simulink model "Enable_Subsystem"  (R2024b)
settings: Solver=VariableStepAuto  StartTime=0.0  StopTime=10.0  RelTol=1e-3
settings Model: Creator=Ahmad  LastModifiedBy=Ahmad

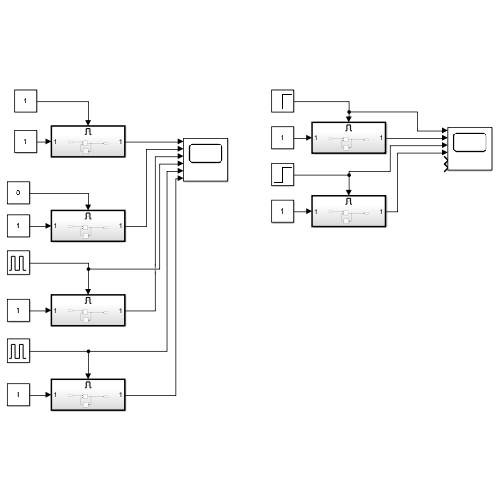
[thumbnail: Simulink's stored preview of the top-level diagram]
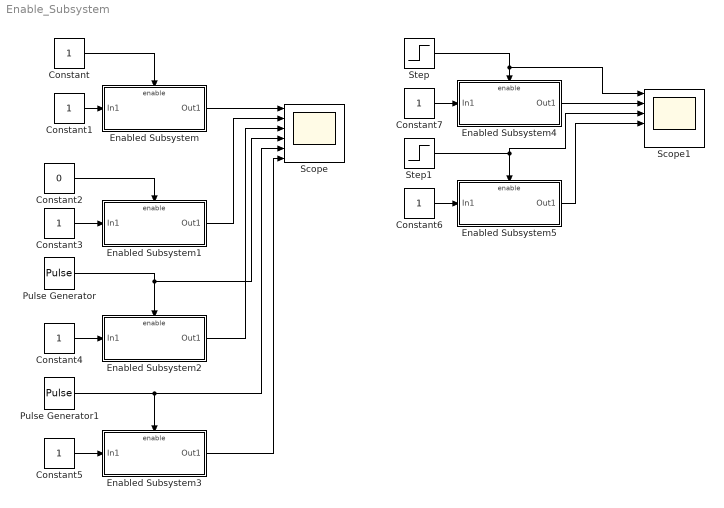
== system Enable_Subsystem ==
  Constant{,1,3..7} (7 alike) : Constant
  Constant2 : Constant  Value=0
  Enabled Subsystem : Subsystem  TreatAsAtomicUnit=on
  Enabled Subsystem1 : Subsystem  TreatAsAtomicUnit=on
  Enabled Subsystem2 : Subsystem  TreatAsAtomicUnit=on
  Enabled Subsystem3 : Subsystem  TreatAsAtomicUnit=on
  Enabled Subsystem4 : Subsystem  TreatAsAtomicUnit=on
  Enabled Subsystem5 : Subsystem  TreatAsAtomicUnit=on
  Pulse Generator : DiscretePulseGenerator  PulseType=Time based  Period=1  PulseWidth=50
  Pulse Generator1 : DiscretePulseGenerator  PulseType=Time based  Period=1  PulseWidth=50
  Scope : Scope  NumInputPorts=6
  Scope1 : Scope  NumInputPorts=6
  Step : Step  SampleTime=0
  Step1 : Step  Before=-2  After=0  SampleTime=0
  wires:
  Enabled Subsystem/1(Out1) -> Scope/1
  Constant/1 -> Enabled Subsystem/Enable
  Constant1/1 -> Enabled Subsystem/1(In1)
  Constant3/1 -> Enabled Subsystem1/1(In1)
  Constant2/1 -> Enabled Subsystem1/Enable
  Enabled Subsystem1/1(Out1) -> Scope/2
  Constant4/1 -> Enabled Subsystem2/1(In1)
  Pulse Generator/1 -> Enabled Subsystem2/Enable, Scope/4
  Enabled Subsystem2/1(Out1) -> Scope/3
  Pulse Generator1/1 -> Scope/5, Enabled Subsystem3/Enable
  Constant5/1 -> Enabled Subsystem3/1(In1)
  Enabled Subsystem3/1(Out1) -> Scope/6
  Constant7/1 -> Enabled Subsystem4/1(In1)
  Step/1 -> Scope1/1, Enabled Subsystem4/Enable
  Enabled Subsystem4/1(Out1) -> Scope1/2
  Constant6/1 -> Enabled Subsystem5/1(In1)
  Step1/1 -> Scope1/3, Enabled Subsystem5/Enable
  Enabled Subsystem5/1(Out1) -> Scope1/4

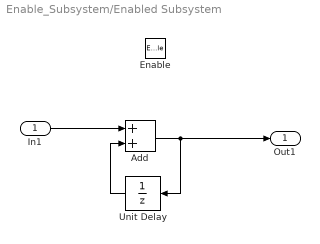
== system Enable_Subsystem/Enabled Subsystem ==
  In1 : Inport
  Enable : EnablePort
  Add : Sum
  Unit Delay : UnitDelay  SampleTime=-1  HasFrameUpgradeWarning=on
  Out1 : Outport
  wires:
  In1/1 -> Add/1
  Add/1 -> Unit Delay/1, Out1/1
  Unit Delay/1 -> Add/2

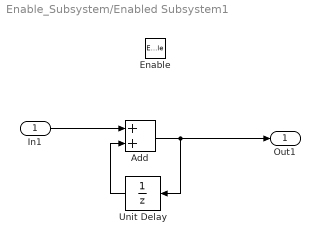
== system Enable_Subsystem/Enabled Subsystem1 ==
  In1 : Inport
  Enable : EnablePort
  Add : Sum
  Unit Delay : UnitDelay  SampleTime=-1  HasFrameUpgradeWarning=on
  Out1 : Outport
  wires:
  In1/1 -> Add/1
  Add/1 -> Unit Delay/1, Out1/1
  Unit Delay/1 -> Add/2

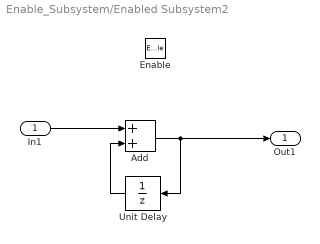
== system Enable_Subsystem/Enabled Subsystem2 ==
  In1 : Inport
  Enable : EnablePort
  Add : Sum
  Unit Delay : UnitDelay  SampleTime=-1  HasFrameUpgradeWarning=on
  Out1 : Outport
  wires:
  In1/1 -> Add/1
  Add/1 -> Unit Delay/1, Out1/1
  Unit Delay/1 -> Add/2

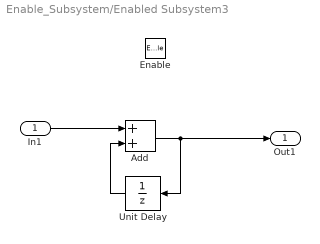
== system Enable_Subsystem/Enabled Subsystem3 ==
  In1 : Inport
  Enable : EnablePort  StatesWhenEnabling=reset
  Add : Sum
  Unit Delay : UnitDelay  SampleTime=-1  HasFrameUpgradeWarning=on
  Out1 : Outport
  wires:
  In1/1 -> Add/1
  Add/1 -> Unit Delay/1, Out1/1
  Unit Delay/1 -> Add/2

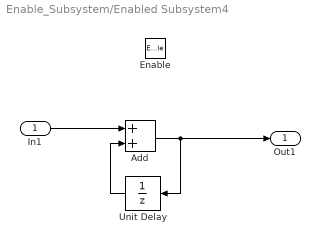
== system Enable_Subsystem/Enabled Subsystem4 ==
  In1 : Inport
  Enable : EnablePort
  Add : Sum
  Unit Delay : UnitDelay  SampleTime=-1  HasFrameUpgradeWarning=on
  Out1 : Outport
  wires:
  In1/1 -> Add/1
  Add/1 -> Unit Delay/1, Out1/1
  Unit Delay/1 -> Add/2

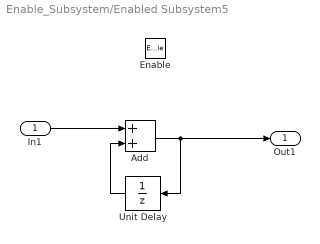
== system Enable_Subsystem/Enabled Subsystem5 ==
  In1 : Inport
  Enable : EnablePort
  Add : Sum
  Unit Delay : UnitDelay  SampleTime=-1  HasFrameUpgradeWarning=on
  Out1 : Outport
  wires:
  In1/1 -> Add/1
  Add/1 -> Unit Delay/1, Out1/1
  Unit Delay/1 -> Add/2
